simulink model "BlockDemo"  (Simulink 6.3)
settings: Solver=FixedStepDiscrete  StartTime=0.0  StopTime=33  RelTol=1e-3
InitFcn:
  | %% DSPBuilder Start
  | alt_dspbuilder_update_model(bdroot)
  | %% DSPBuilder End
libraries: allblocks_alteradspbuilder2 x9
settings Model: Creator=mjervis  LastModifiedBy=delphick
settings OptimizationCC: BlockReduction=off  BooleanDataType=off  InlineInvariantSignals=on
settings DebuggingCC: SolverPrmCheckMsg=none
settings HardwareCC: TargetUnknown=on

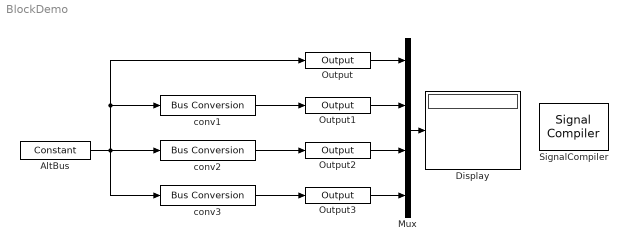
== system BlockDemo ==
  AltBus : allblocks_alteradspbuilder2/Constant  mask_cst=-127.625  BusType=Signed Fractional  bwl=10  bwr=10  SpecifyClock=off
  Display : Display
  Mux : Mux
  Output : allblocks_alteradspbuilder2/Output  iofile=C:\workspace_clean\Documentation\DesignExamples\Tutorials\UnitBlocks\IOBus\BusConversion\tb_BlockDemo\BlockDemo_Output.capture  BusType=Inferred  bwl=10  bwr=10  PORTTYPE=Output
  Output1 : allblocks_alteradspbuilder2/Output  iofile=C:\workspace_clean\Documentation\DesignExamples\Tutorials\UnitBlocks\IOBus\BusConversion\tb_BlockDemo\BlockDemo_Output1.capture  BusType=Inferred  bwl=10  bwr=2  PORTTYPE=Output
  Output2 : allblocks_alteradspbuilder2/Output  iofile=C:\workspace_clean\Documentation\DesignExamples\Tutorials\UnitBlocks\IOBus\BusConversion\tb_BlockDemo\BlockDemo_Output2.capture  BusType=Inferred  bwl=4  bwr=0  PORTTYPE=Output
  Output3 : allblocks_alteradspbuilder2/Output  iofile=C:\workspace_clean\Documentation\DesignExamples\Tutorials\UnitBlocks\IOBus\BusConversion\tb_BlockDemo\BlockDemo_Output3.capture  BusType=Inferred  bwl=8  bwr=0  PORTTYPE=Output
  SignalCompiler : allblocks_alteradspbuilder2/Signal Compiler  DeviceFamily=Stratix IV  DeviceName=AUTO  EnableSignalTap=off  SignalTapDepth=128  UseBoardBlock=off  StpUseDefaultClock=on  StpClock=clock
  conv1 : allblocks_alteradspbuilder2/Bus Conversion  BusType=Signed Fractional  ibwl=10  ibwr=10  bwl=8  bwr=2  bitToConnectToOutputLSB=1  round=off  saturate=on
  conv2 : allblocks_alteradspbuilder2/Bus Conversion  BusType=Signed Fractional  ibwl=10  ibwr=10  bwl=8  bwr=1  bitToConnectToOutputLSB=0  round=on  saturate=off
  conv3 : allblocks_alteradspbuilder2/Bus Conversion  BusType=Signed Integer  ibwl=20  ibwr=10  bwl=10  bwr=2  bitToConnectToOutputLSB=0  round=off  saturate=off
  wires:
  AltBus/1 -> conv1/1, Output/1, conv2/1, conv3/1
  conv1/1 -> Output1/1
  conv2/1 -> Output2/1
  conv3/1 -> Output3/1
  Mux/1 -> Display/1
  Output/1 -> Mux/1
  Output1/1 -> Mux/2
  Output2/1 -> Mux/3
  Output3/1 -> Mux/4
